simulink library "PhD_Library"  (R2018a)
settings: Solver=VariableStepAuto  StartTime=0.0  StopTime=10.0  RelTol=1e-3
values from neighbouring files (symbols this model uses):
  fn = 60    [Basics_01_Param.m]    (also in FIRs.m = 50; PostSubmission_FreqResp_00_Param.m; XoverRCalc.m)
  Ts_control = 1/20000    (= 5e-05)    [Basics_01_Param.m]    (also in PostSubmission_FreqResp_00_Param.m)
  Ts_PWM = 1/200000    (= 5e-06)    [Basics_01_Param.m]    (also in PostSubmission_FreqResp_00_Param.m)
  Uanp = 1    [Basics_01_Param.m]    (also in PostSubmission_FreqResp_00_Param.m)
undefined symbols (not defined in the file or in its folder): D1, Delta, DiscIntNeverNeededParam, ESS, Iap, PCC, Sn, tctrl, WT
libraries: $bdroot x49, powerlib_meascontrol x39, peTransforms x28, powerlib x18
(part 1 of 3)
settings Model: Creator=daniemot  LastModifiedBy=daniemot

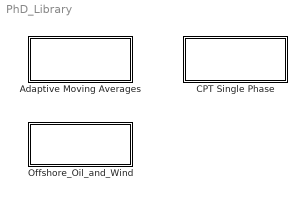
== system PhD_Library ==
  Adaptive Moving Averages : Subsystem
  CPT Single Phase : Subsystem
  Offshore_Oil_and_Wind : Subsystem

== system PhD_Library/Adaptive Moving Averages ==
  AMA with insertion pointer driven buffer : Subsystem  TreatAsAtomicUnit=on  SystemSampleTime=Ts  mask(AMA with insertion pointer driven){NbSize=100, Ts=0.001}
      mask prompts: NbSize "Max number of samples for averaging"; Ts "Sampling time [s]"
      mask help:
      | Adaptive moving average with insertion pointer driven circular buffer
      |
      | Interface
      | Input	x (scalar): signal for averaging
      | 	n (scalar): number of previous samples of the input to be averaged with the current input
      | Output	xavg (scalar): average of the current input and the last n-samples of the input.
      | 	xacc (scalar): internal value sent for accumulation
      | 	xdec (scalar): internal value sent for decumulation
      | Parameters	nmax (scalar): maximum length of the length of the circular buffer
      | 	Ts (scalar): sampling time in [s]
      | Internal circular buffer:
      | 	Insertion pointer: i, always marches forward, x(now) replaces the slot pointed by i
      | 	Retrieval pointer: r, lags i by n samples, zeros the slot once retrieved, allowed to jump backwards, collects all values for decumulation and zeros slots when jumping forward.
      |
      | Prog/rev. semi-history:
      | 	Mota, 2020-11-24: first release
  AMA with lossy buffer : Subsystem  TreatAsAtomicUnit=on  SystemSampleTime=Ts  mask(AMA with a skipping circular buffer.){NbSize=100, Ts=0.001}
      mask prompts: NbSize "Max number of samples for averaging"; Ts "Sampling time [s]"
      mask help:
      | Adaptive moving average built with Matlab's discrete variable time delay
      |
      | Interface
      | Input	x (scalar): signal for averaging
      | 	n (scalar): number of previous samples of the input to be averaged with the current input
      | Output	xavg (scalar): average of the current input and the last n-samples of the input.
      | 	xacc (scalar): internal value sent for accumulation
      | 	xdec (scalar): internal value sent for decumulation
      | Parameters	nmax (scalar): maximum length of the length of the circular buffer
      | 	Ts (scalar): sampling time in [s]
      | Internal circular buffer:
      | 	Matlab's variable discrete time delay
      | 	Skips/double decumulations when n changes
      |
      | Prog/rev. semi-history:
      | 	Mota, 2020-11-24: first release
  AMA with retrieval pointer driven buffer : Subsystem  TreatAsAtomicUnit=on  SystemSampleTime=Ts  mask(AMA with retrieval pointer driven buffer){NbSize=100, Ts=0.001}
      mask prompts: NbSize "Max number of samples for averaging"; Ts "Sampling time [s]"
      mask help:
      | Adaptive moving average with retrieval poitner driven circular buffer
      |
      | Interface
      | Input	x (scalar): signal for averaging
      | 	n (scalar): number of previous samples of the input to be averaged with the current input
      | Output	xavg (scalar): average of the current input and the last n-samples of the input.
      | 	xacc (scalar): internal value sent for accumulation
      | 	xdec (scalar): internal value sent for decumulation
      | Parameters	nmax (scalar): maximum length of the length of the circular buffer
      | 	Ts (scalar): sampling time in [s]
      | Internal circular buffer:
      | 	Retrieval pointer: r, always marches forward, zero the slot after retrieval.
      | 	Insertion pointer: i, marches n slots ahead of r, allowed to jump, sums x(now) to the whichever value present at the insertion slot
      |
      | Prog/rev. semi-history:
      | 	Mota, 2020-11-24: first release
  Subsystem : Subsystem  TreatAsAtomicUnit=on  SystemSampleTime=Ts  mask(HAMA with retrieval pointer driven buffer){NbSize=100, Ts=0.001}
      mask prompts: NbSize "Max number of samples for averaging"; Ts "Sampling time [s]"
      mask help:
      | Hybrid adaptive moving average with three retrieval pointer driven circular buffers.
      |
      | Interface
      | Input	x (scalar): signal for averaging
      | 	n (scalar): number of previous samples of the input to be averaged with the current input
      | Output	xavg (scalar): average of the current input and the last hybrid number of 'n'-samples of the input.
      | 	xavground (scalar): average of the current input and the last round(n)-samples of the input.
      | 	xavgceil (scalar): average of the current input and the last ceil(n)-samples of the input.
      | 	xavgfloor (scalar): average of the current input and the last floor(n)-samples of the input.
      | 	xavgweighed (scalar): average of the current input and the last weighted(n)-samples of the input.
      | Parameters	nmax (scalar): maximum length of the length of the circular buffer
      | 	Ts (scalar): sampling time in [s]
      |
      | Prog/rev. semi-history:
      | 	Mota, 2020-12-08: first release
  WAMA with insertion pointer driven buffer : Subsystem  TreatAsAtomicUnit=on  SystemSampleTime=Ts  mask(WAMA with insertion pointer driven buffer){NbSize=0, Ts=0}
      mask prompts: NbSize "Max number of samples for averaging"; Ts "Sampling time [s]"
      mask help:
      | Adaptive moving average with two insertion pointer driven circular buffers.
      |
      | Interface
      | Input	x (scalar): signal for averaging
      | 	n (scalar): number of previous samples of the input to be averaged with the current input
      | Output	xavg (scalar): weigthed average of the current input and the last 'n'-samples of the input.
      | 	xavgceil (scalar): average of the current input and the last ceil(n)-samples of the input.
      | 	xavgfloor (scalar): average of the current input and the last floor(n)-samples of the input.
      | Parameters	nmax (scalar): maximum length of the length of the circular buffer
      | 	Ts (scalar): sampling time in [s]
      |
      | Prog/rev. semi-history:
      | 	Mota, 2020-11-24: first release
  WAMA with retrieval pointer driven buffers : Subsystem  TreatAsAtomicUnit=on  SystemSampleTime=Ts  mask(WAMA with retrieval pointer driven buffer){NbSize=100, Ts=0.001}
      mask prompts: NbSize "Max number of samples for averaging"; Ts "Sampling time [s]"
      mask help:
      | Adaptive moving average with two retrieval pointer driven circular buffers.
      |
      | Interface
      | Input	x (scalar): signal for averaging
      | 	n (scalar): number of previous samples of the input to be averaged with the current input
      | Output	xavg (scalar): weigthed average of the current input and the last 'n'-samples of the input.
      | 	xavgceil (scalar): average of the current input and the last ceil(n)-samples of the input.
      | 	xavgfloor (scalar): average of the current input and the last floor(n)-samples of the input.
      | Parameters	nmax (scalar): maximum length of the length of the circular buffer
      | 	Ts (scalar): sampling time in [s]
      |
      | Prog/rev. semi-history:
      | 	Mota, 2020-11-24: first release

== system PhD_Library/CPT Single Phase ==
  Single phase CPT Lossy AMA : Subsystem  TreatAsAtomicUnit=on  SystemSampleTime=Ts  mask(Single phase CPT transducer with Skipping AMAs){NbSize=100, Ts=0.001}
      mask prompts: NbSize "Maximum number of samples per period"; Ts "Sampling time [s]"
      mask help:
      | Input	Voltage: v, scalar
      | 	Current: i, scalar
      | 	Frequecy: f, scalar in [Hz]
      | Output	Active power: p
      | 	Active current: ia
      | 	Reactive power: q
      | 	Reactive energy: w
      | 	Reactive current: ir
      | 	Void current: iv
      | 	Integral of the voltage: vint
      | 	Bias of the int. of the volt.: vintbias
      | 	Voltage times current: vi
      | 	Unbiased int. voltage times current: vinthati
      | Parameters	nmax (scalar): maximum length of the length of the circular buffers
      | 	Ts (scalar): sampling time in [s]
      |
      | Prog/rev. semi-history:
      | 	Mota, 2020-11-24: first release
      | 	Mota, 2020-12-08: added voltages and currents to interface
  Single phase CPT Retrieval AMA : Subsystem  TreatAsAtomicUnit=on  SystemSampleTime=Ts  mask(Single Phase CPT Retrieval AMAs){NbSize=100, Ts=0.001}
      mask prompts: NbSize "Maximum number of samples per period"; Ts "Sampling time [s]"
      mask help:
      | Input	Voltage: v, scalar
      | 	Current: i, scalar
      | 	Frequecy: f, scalar in [Hz]
      | Output	Active power: p
      | 	Active current: ia
      | 	Reactive power: q
      | 	Reactive energy: w
      | 	Reactive current: ir
      | 	Void current: iv
      | 	Integral of the voltage: vint
      | 	Bias of the int. of the volt.: vintbias
      | 	Voltage times current: vi
      | 	Unbiased int. voltage times current: vinthati
      | Parameters	nmax (scalar): maximum length of the length of the circular buffers
      | 	Ts (scalar): sampling time in [s]
      |
      | Prog/rev. semi-history:
      | 	Mota, 2020-11-24: first release
      | 	Mota, 2020-12-08: added voltages and currents to interface
  Single phase CPT Retrieval HAMA : Subsystem  TreatAsAtomicUnit=on  SystemSampleTime=Ts  mask{NbSize=100, Ts=0.001}
      mask prompts: NbSize "Maximum number of samples per period"; Ts "Sampling time [s]"
      mask help:
      | Input	Voltage: v, scalar
      | 	Current: i, scalar
      | 	Frequecy: f, scalar in [Hz]
      | Output	Active power: p
      | 	Active current: ia
      | 	Reactive power: q
      | 	Reactive energy: w
      | 	Reactive current: ir
      | 	Void current: iv
      | 	Integral of the voltage: vint
      | 	Bias of the int. of the volt.: vintbias
      | 	Voltage times current: vi
      | 	Unbiased int. voltage times current: vinthati
      | Parameters	nmax (scalar): maximum length of the length of the circular buffers
      | 	Ts (scalar): sampling time in [s]
      |
      | Prog/rev. semi-history:
      | 	Mota, 2020-12-08: first release
  Single phase CPT Retrieval WAMA : Subsystem  TreatAsAtomicUnit=on  SystemSampleTime=Ts  mask(Single phase CPT with Retrieval WAMAs){NbSize=100, Ts=0.001}
      mask prompts: NbSize "Maximum number of samples per period"; Ts "Sampling time [s]"
      mask help:
      | Input	Voltage: v, scalar
      | 	Current: i, scalar
      | 	Frequecy: f, scalar in [Hz]
      | Output	Active power: p
      | 	Active current: ia
      | 	Reactive power: q
      | 	Reactive energy: w
      | 	Reactive current: ir
      | 	Void current: iv
      | 	Integral of the voltage: vint
      | 	Bias of the int. of the volt.: vintbias
      | 	Voltage times current: vi
      | 	Unbiased int. voltage times current: vinthati
      | Parameters	nmax (scalar): maximum length of the length of the circular buffers
      | 	Ts (scalar): sampling time in [s]
      |
      | Prog/rev. semi-history:
      | 	Mota, 2020-11-24: first release
      | 	Mota, 2020-12-08: added voltages and currents to interface

== system PhD_Library/Offshore_Oil_and_Wind ==
  note: WILL MOST LIKELY BE ABANDONED
  Balanced_3_phase_Vsource : Subsystem  mask(Three-phase ideal voltage source){BaseAmp=1, fn=50}
      mask prompts: BaseAmp "Base phase-to-neutral amplitude [V]"; fn "Base frequency [Hz]"
      mask help:
      | Three-phase balanced ideal voltage source with neutral point not connected.
      | The voltage source can be connected in series with others.
      |
      | va [V] = amp_pu*BaseAmp*sin(2*pi*f_pu*fn*time + phase_deg*pi/180)
      | vb [V] = amp_pu*BaseAmp*sin(2*pi*f_pu*fn*time + phase_deg*pi/180 + Ph_b_sign*2*pi/3)
      | vc [V] = amp_pu*BaseAmp*sin(2*pi*f_pu*fn*time + phase_deg*pi/180 + Ph_c_sign*2*pi/3)
      |
      | If Pos1_Neg-1 = 1
      | 	Ph_b_sign = -1
      | 	Ph_c_sign = +1
      |
      | If Pos1_Neg-1 = -1
      | 	Ph_b_sign = +1
      | 	Ph_c_sign = -1
  Digital first order LPF : Subsystem  mask(Digital first order low pass filter){Ts=tctrl, fcutout=fn/2^0.5}
      mask prompts: Ts "Sample times [s]"; fcutout "Cutout frequency [Hz]"
      mask help:
      | Integration with trapezoidal approximation.
      |
      | "Continuous time transfer function":  1/(1 + s T)
      | where T [s] = 1 / (2 * pi * fcutout [Hz]).
      mask Display: fprintf('1/(1 + s T))');
  Idq_Controller : Subsystem  mask(Idq Controller - PI regulator with anti-windup){Ts=Ts_control, fn=fn, Kp=0.4, Ti=0.13, I_ini_d=0.14, I_ini_q=0.07, L=WT.LSC.lf1, PI_max=1.5, PI_min=-1.5, TrafoPhaseComp=0}
      mask prompts: Ts "Sampling time [s]"; fn "Rated frequency: fn [Hz]"; Kp "Proportional gain: Kp [pu]"; Ti "Integral time: Ti [s]"; I_ini_d "Initial value for D integrator [pu]"; I_ini_q "Initial value for Q integrator [pu]"; L "DQ decoupl. inductance: L [pu]"; PI_max "Maximum output [pu]"; PI_min "Minimum output [pu]"; TrafoPhaseComp "Transformer phase compensation [rad]"
      mask help:
      | Idq Controller
      | Discrete PI regulator with forward Euler approximation for the integrator.
      | Transfer function: 	Kp (1 + sTi) / (sTi)
      | The anti-windup freezes the integrator if the unlimited output of the PI goes beyond the limits.
      |
      | Phase compensation for transformer winding: PhaseTrafoComp
  Idq_Decouling_Signs : Subsystem  mask(Idq Controller - PI regulator with anti-windup){Ts=Ts_control, fn=50, Kp=0.4, Ti=0.13, I_ini_d=0.14, I_ini_q=0.07, L=0.3, PI_max=1.5, PI_min=-1.5, TrafoPhaseComp=0}
      mask prompts: Ts "Sampling time [s]"; fn "Rated frequency: fn [Hz]"; Kp "Proportional gain: Kp [pu]"; Ti "Integral time: Ti [s]"; I_ini_d "Initial value for D integrator [pu]"; I_ini_q "Initial value for Q integrator [pu]"; L "DQ decoupl. inductance: L [pu]"; PI_max "Maximum output [pu]"; PI_min "Minimum output [pu]"; TrafoPhaseComp "Transformer phase compensation [rad]"
      mask help:
      | Idq Controller
      | Discrete PI regulator with forward Euler approximation for the integrator.
      | Transfer function: 	Kp (1 + sTi) / (sTi)
      | The anti-windup freezes the integrator if the unlimited output of the PI goes beyond the limits.
      |
      | Phase compensation for transformer winding: PhaseTrafoComp
  LSC_LCL_Trafo : Subsystem  mask(LSC + LCL + Trafo){Sn=WT.Sb, fn=fn, Uhv_ab=WT.ColSys.Ub, Uab=WT.LSC.Ub, lf2=WT.LSC.lf2, rf2=WT.LSC.rf2, Lf1=WT.LSC.Lf1, Rf1=WT.LSC.Rf1, Cf=WT.LSC.Cf, Rc=WT.LSC.Rc}
      mask prompts: Sn "Rated apparent power [VA]"; fn "Rated frequency [Hz]"; Uhv_ab "Trafo HV rated line voltage [V]"; Uab "Trafo LV rated line voltage [V]"; lf2 "Trafo short-circuit inductance, lf2 [pu]"; rf2 "Trafo short-circuit resistance, rf2 [pu]"; Lf1 "Inverter side inductande, Lf1 [H]"; Rf1 "Inverter side parasitic resistance, Rf1 [Ohm]"; Cf "Shunt branch capacitance, Cf [F]"; Rc "Shunt branch damping resistance, Rc [Ohm]"
      mask help:
      | Line side converter + LCL filter + Transformer
      |
      | LSC: switching devices
      | LCL:
      | 	Lf1 + Rf1: inverter side reactor
      | 	Cf + Rc: shunt capacitor and damping resistor
      | 	Lf2 + Rf2: transformer short circuit inductance and resistance
      |
      | Transformer:	Y d1
      | 	HV: Y ungrounded
      | 	LV: delta
      |
      | High resistive grounding on LV side of tranformer (0.001W)
  PI_Kp_Ti_AntiWindup : Subsystem  TreatAsAtomicUnit=on  SystemSampleTime=Ts  mask(PI regulator with anti-windup){Ts=0.001, Kp=10, Ti=1, I_ini=0, PI_max=1, PI_min=-1}
      mask prompts: Ts "Sampling time [s]"; Kp "Proportional gain: Kp [pu]"; Ti "Integral time: Ti [s]"; I_ini "Initial value for the integrator [pu]"; PI_max "Maximum output [pu]"; PI_min "Minimum output [pu]"
      mask help:
      | Discrete PI regulator with forward Euler approximation for the integrator.
      |
      | Transfer function:
      | 	Kp (1 + sTi) / (sTi)
      |
      | The anti-windup freezes the integrator if the unlimited output of the PI goes beyond the limits.
      mask Display: fprintf('Kp(1+1/(sTi))');
  PLL : Subsystem  mask(Matlabs PLL with POS and NEG omega t output){fn=0, Ts=0.00005, Kp_pll=90, Ki_pll=1600, Kd_pll=0, PLL_ini=0}
      mask prompts: fn "Rated frequency [Hz]"; Ts "Sampling time [s]"; Kp_pll "Proportional gain: Kp_pll"; Ki_pll "Integral gain: Ki_pll"; Kd_pll "Derivative gain: Kd_pll"; PLL_ini "PLL initial angle: PLL_ini [degrees]"
  PWM : Subsystem  mask(Scaling of vdq ref and PWM gate generation){fsw=0, Ts=1/200000, Uabp=1000, PWM_Ini_Phase=90}
      mask prompts: fsw "Switching frequency [Hz]"; Ts "Sampling time [s]"; Uabp "Rated peak line voltage [V]"; PWM_Ini_Phase "PWM carrier initial phase [degrees]"
      mask help:
      | Scales vdq_ref by: U_line_peak / Udc
      |
      | Add third harmonic to uabc_ref for overmodulation
  PWM_abc_negwt_acb : Subsystem  mask(Scaling of vdq ref and PWM gate generation){fsw=50, Ts=1/200000, Uabp=1000, PWM_Ini_Phase=90}
      mask prompts: fsw "Switching frequency [Hz]"; Ts "Sampling time [s]"; Uabp "Rated peak line voltage [V]"; PWM_Ini_Phase "PWM carrier initial phase [degrees]"
      mask help:
      | Scales vdq_ref by: U_line_peak / Udc
      |
      | Add third harmonic to uabc_ref for overmodulation
  Scaling_and_PWM : Subsystem  mask(Scaling of vdq ref and PWM gate generation){Ts=Ts_PWM, Uabp=1000, PWM_Ini_Phase=90}
      mask prompts: Ts "Sampling time [s]"; Uabp "Rated peak line voltage [V]"; PWM_Ini_Phase "PWM carrier initial phase [degrees]"
      mask help:
      | Scales vdq_ref by: U_line_peak / Udc
      |
      | Add third harmonic to uabc_ref for overmodulation
  Udc_Controller : Subsystem  mask(Udc Controller - PI regulator with anti-windup){Ts=Ts_control, Kp=WT.LSC.Kp, Ti=WT.LSC.Ti, I_ini=0, PI_max=1.5, PI_min=-1.5}
      mask prompts: Ts "Sampling time [s]"; Kp "Proportional gain: Kp [pu]"; Ti "Integral time: Ti [s]"; I_ini "Initial value for integrator [pu]"; PI_max "Maximum output [pu]"; PI_min "Minimum output [pu]"
      mask help:
      | Udc Controller
      | Discrete PI regulator with forward Euler approximation for the integrator.
      | Transfer function: 	Kp (1 + sTi) / (sTi)
      | The anti-windup freezes the integrator if the unlimited output of the PI goes beyond the limits.
  abc-dq_DDSRF_PLL_Based : Subsystem  mask(abc -> dq based on DDSRF PLL){Ts=Ts_control, fc=fn/2^0.5}
      mask prompts: Ts "Sampling time [s]"; fc "Cutout freq. low pass [Hz]"
      mask help:
      | abc -> dq transducer based on the Decoupled Double Synchronous Reference Frame PLL for Power Converters Control from Rodriguez 2007.
      | The PLL is not implemented, but an output with eq is available for using in a PLL
  abc_dq : Subsystem  mask(abc->dq with Matlab){Ts=0.001, fn=100, fcutoutv=1000, fcutouti=1000, zeta=0.707}
      mask prompts: Ts "Sampling time [s]"; fn "Notch frequency [Hz]"; fcutoutv "Cutout freq. low-pass for vdq meas. [Hz]"; fcutouti "Cutout freq. low-pass for idq meas. [Hz]"; zeta "Zeta for notch filters"
  abc_dq_Rodriguez : Subsystem  mask(abc - dq with double decopupling){Ts=0.00001, fcutout=50/2^0.5}
      mask prompts: Ts "Sampling time [s]"; fcutout "Cutout freq. low pass [Hz]"
      mask help:
      | Double decoupling - Rodriguez
      |
      | The PLL is not implemented, but an output with eq is available for using in a PLL
  abc_dq_with_AMA : Subsystem  mask(abc->dq with Matlab){Ts=0.001, fn=100, fmin=0, fmax=0, fcutoutv=1000, fcutouti=1000}
      mask prompts: Ts "Sampling time [s]"; fn "Rated grid frequency [Hz]"; fmin "Min. acceptable grid freq [Hz]"; fmax "Max. acceptable grid freq [Hz]"; fcutoutv "Cutout freq. low-pass for vdq meas. [Hz]"; fcutouti "Cutout freq. low-pass for idq meas. [Hz]"
  abc_dq_with_PLL : Subsystem  mask(abc->dq with Matlab){Ts=0.001, Kp_pll=90, Ki_pll=1600, Kd_pll=0, PLL_ini=0, fn=50, fcutoutv=1000, fcutouti=1000, zeta=0.7}
      mask prompts: Ts "Sampling time [s]"; Kp_pll "Proportional gain: Kp_pll"; Ki_pll "Integral gain: Ki_pll"; Kd_pll "Derivative gain: Kd_pll"; PLL_ini "PLL initial angle: PLL_ini [degrees]"; fn "Notch frequency [Hz]"; fcutoutv "Cutout freq. low-pass for vdq meas. [Hz]"; fcutouti "Cutout freq. low-pass for idq meas. [Hz]"; zeta "Zeta for all second order filters"
  pqui_Transd_NoZeroSeq : Subsystem  mask(u i p q transducer - No zero sequence){Sn=Sn, Uanp=Uanp, Iap=Iap}
      mask prompts: Sn "Rated three-phase apparent power [VA]"; Uanp "Rated peak phase-to-groud voltage [V]"; Iap "Rated peak line current [A]"
      mask help:
      | Loosely based on Akagi 1984, but with Clarke Transformation for both the current and voltage
      | 	v  = (valpha^2 + vbeta^2)^0.5 / V_phase_peak
      | 	i   = (ialpha^2 + ibeta^2)^0.5 / I_line_peak
      | 	p  = 3/2 * (valpha ialpha +vbeta ibeta) / Sn
      | 	q  = 3/2 * (-valpha ibeta +vbeta ialpha) / Sn
  pqui_Transd_NoZeroSeq_Filter : Subsystem  mask(u i p q transducer - No zero sequence){Ts=0.001, Sn=1000, fn=50, Uanp=1000, Iap=1000, fcutoutvi=1000, fcutoutpq=1000, zeta=0.7}
      mask prompts: Ts "Sampling time [s]"; Sn "Rated three-phase apparent power [VA]"; fn "Rated frequency [Hz]"; Uanp "Rated peak phase-to-groud voltage [V]"; Iap "Rated peak line current [A]"; fcutoutvi "Cutout freq. low-pass for v&i meas. [Hz]"; fcutoutpq "Cutout freq. low-pass for p&q meas. [Hz]"; zeta "Zeta for all second order filters"
      mask help:
      | Loosely based on Akagi 1984, but with Clarke Transformation for both the current and voltage
      | 	v  = (valpha^2 + vbeta^2)^0.5 / V_phase_peak
      | 	i   = (ialpha^2 + ibeta^2)^0.5 / I_line_peak
      | 	p  = 3/2 * (valpha ialpha +vbeta ibeta) / Sn
      | 	q  = 3/2 * (-valpha ibeta +vbeta ialpha) / Sn
      |
      | Second order low-pass filter for all measurements
      |
      | Notch filter at the rated frequency

== system PhD_Library/Adaptive Moving Averages/AMA with insertion pointer driven buffer ==
  In1 : Inport
  In2 : Inport  Port=2
  Constant3 : Constant  Value=NbSize
  MATLAB Function : MATLAB Function  TreatAsAtomicUnit=on
  Out1 : Outport
  Out2 : Outport  Port=2
  Out3 : Outport  Port=3
  wires:
  In2/1 -> MATLAB Function/2(n)  "n"
  MATLAB Function/1(xavg) -> Out1/1  "xavg"
  Constant3/1 -> MATLAB Function/3(Nb)
  MATLAB Function/2(xacc) -> Out2/1  "xacc"
  MATLAB Function/3(xdec) -> Out3/1  "xdec"
  In1/1 -> MATLAB Function/1(x)  "x"

== system PhD_Library/Adaptive Moving Averages/AMA with lossy buffer ==
  x : Inport
  n : Inport  Port=2
  Add1 : Sum
  Add4 : Sum  Inputs=+-
  Constant : Constant
  Delay2 : Delay  DelayLength=1  InitialCondition=0  UseCircularBuffer=on  SampleTime=Ts
  Divide1 : Product  Inputs=*/
  Max : MinMax  Function=max  Inputs=2
  Rounding Function : Rounding  Operator=round
  Variable Integer Delay2 : Delay  DelayLengthSource=Input port  DelayLengthUpperLimit=NbSize  UseCircularBuffer=on  SampleTime=Ts
      settings: InputPortMap=u0,p1
  Zero-Order Hold : ZeroOrderHold  Commented=through  SampleTime=Ts
  Zero-Order Hold1 : ZeroOrderHold  Commented=through  SampleTime=Ts
  xavg : Outport
  xacc : Outport  Port=2
  xdec : Outport  Port=3
  wires:
  n/1 -> Zero-Order Hold1/1  "n"
  x/1 -> Zero-Order Hold/1  "x"
  Divide1/1 -> Add4/1, Variable Integer Delay2/1, xacc/1  "xacc"
  Variable Integer Delay2/1 -> Add4/2, xdec/1  "xdec"
  Constant/1 -> Max/2
  Max/1 -> Variable Integer Delay2/2  "n"
  Add4/1 -> Add1/1  "xavg"
  Add1/1 -> Delay2/1, xavg/1  "xavg"
  Delay2/1 -> Add1/2
  Zero-Order Hold/1 -> Divide1/1
  Zero-Order Hold1/1 -> Rounding Function/1
  Rounding Function/1 -> Divide1/2, Max/1

== system PhD_Library/Adaptive Moving Averages/AMA with retrieval pointer driven buffer ==
  In1 : Inport
  In2 : Inport  Port=2
  Constant3 : Constant  Value=NbSize
  MATLAB Function : MATLAB Function  TreatAsAtomicUnit=on
  Out1 : Outport
  Out2 : Outport  Port=2
  Out3 : Outport  Port=3
  wires:
  MATLAB Function/3(xdec) -> Out3/1  "xdec"
  MATLAB Function/1(xavg) -> Out1/1  "xavg"
  Constant3/1 -> MATLAB Function/3(Nb)
  In1/1 -> MATLAB Function/1(x)  "x"
  In2/1 -> MATLAB Function/2(n)  "n"
  MATLAB Function/2(xacc) -> Out2/1  "xacc"

== system PhD_Library/Adaptive Moving Averages/Subsystem ==
  In1 : Inport
  In2 : Inport  Port=2
  Constant3 : Constant  Value=NbSize
  MATLAB Function : MATLAB Function  TreatAsAtomicUnit=on
  Terminator{,1..3} (4 alike) : Terminator
  Out1 : Outport
  Out3 : Outport  Port=2
  Out4 : Outport  Port=3
  Out2 : Outport  Port=4
  Out5 : Outport  Port=5
  wires:
  MATLAB Function/1(xavg) -> Out1/1  "xavg"
  MATLAB Function/2(xavground) -> Out3/1  "xavground"
  MATLAB Function/3(xavgceil) -> Out4/1  "xavgceil"
  MATLAB Function/4(xavgfloor) -> Out2/1  "xavgfloor"
  MATLAB Function/6(nr) -> Terminator/1  "nr"
  MATLAB Function/7(nf) -> Terminator1/1  "nf"
  MATLAB Function/8(nc) -> Terminator2/1  "nc"
  MATLAB Function/9(changecnt) -> Terminator3/1  "changenc"
  In1/1 -> MATLAB Function/1(x)  "x"
  Constant3/1 -> MATLAB Function/3(Nb)
  In2/1 -> MATLAB Function/2(n)  "n"
  MATLAB Function/5(xavgweigthed) -> Out5/1  "xavgw"

== system PhD_Library/Adaptive Moving Averages/WAMA with insertion pointer driven buffer ==
  In1 : Inport
  In2 : Inport  Port=2
  AMA with insertion pointer driven buffer : $bdroot/Adaptive Moving Averages/AMA with insertion pointer driven buffer  NbSize=NbSize  Ts=Ts
  AMA with insertion pointer driven buffer1 : $bdroot/Adaptive Moving Averages/AMA with insertion pointer driven buffer  NbSize=NbSize  Ts=Ts
  Add : Sum
  Constant : Constant
  Constant1 : Constant
  Floor : Rounding  Operator=ceil
  Floor1 : Rounding
  Max : MinMax  Function=max  Inputs=2
  Product : Product
  Product1 : Product
  Subtract : Sum  Inputs=+-
  Subtract1 : Sum  Inputs=+-+
  Terminator{,1..3} (4 alike) : Terminator
  Out1 : Outport
  Out2 : Outport  Port=2
  Out3 : Outport  Port=3
  wires:
  AMA with insertion pointer driven buffer/1 -> Out2/1, Product/1  "xavgceil"
  AMA with insertion pointer driven buffer/2 -> Terminator/1
  Floor1/1 -> AMA with insertion pointer driven buffer1/2, Subtract1/3, Subtract/2
  Product1/1 -> Add/2
  Subtract/1 -> Product/2
  Product/1 -> Add/1
  Add/1 -> Out1/1  "xavg"
  Subtract1/1 -> Product1/1
  AMA with insertion pointer driven buffer1/2 -> Terminator2/1
  AMA with insertion pointer driven buffer1/3 -> Terminator3/1
  Floor/1 -> AMA with insertion pointer driven buffer/2
  AMA with insertion pointer driven buffer1/1 -> Product1/2, Out3/1  "xavgfloor"
  AMA with insertion pointer driven buffer/3 -> Terminator1/1
  Constant1/1 -> Max/2
  Max/1 -> Floor1/1, Subtract1/2, Subtract/1, Floor/1
  In2/1 -> Max/1  "n"
  Constant/1 -> Subtract1/1
  In1/1 -> AMA with insertion pointer driven buffer1/1, AMA with insertion pointer driven buffer/1  "x"

== system PhD_Library/Adaptive Moving Averages/WAMA with retrieval pointer driven buffers ==
  In1 : Inport
  In2 : Inport  Port=2
  AMA with retrieval pointer driven buffer : $bdroot/Adaptive Moving Averages/AMA with retrieval pointer driven buffer  NbSize=NbSize  Ts=Ts
  AMA with retrieval pointer driven buffer1 : $bdroot/Adaptive Moving Averages/AMA with retrieval pointer driven buffer  NbSize=NbSize  Ts=Ts
  Add : Sum
  Constant : Constant
  Constant1 : Constant
  Floor : Rounding  Operator=ceil
  Floor1 : Rounding
  Max : MinMax  Function=max  Inputs=2
  Product : Product
  Product1 : Product
  Subtract : Sum  Inputs=+-
  Subtract1 : Sum  Inputs=+-+
  Terminator{,1..3} (4 alike) : Terminator
  Out1 : Outport
  Out2 : Outport  Port=2
  Out3 : Outport  Port=3
  wires:
  AMA with retrieval pointer driven buffer/3 -> Terminator1/1
  In1/1 -> AMA with retrieval pointer driven buffer1/1, AMA with retrieval pointer driven buffer/1  "x"
  Floor1/1 -> AMA with retrieval pointer driven buffer1/2, Subtract1/3, Subtract/2
  AMA with retrieval pointer driven buffer/2 -> Terminator/1
  Product1/1 -> Add/2
  Subtract1/1 -> Product1/1
  Add/1 -> Out1/1  "xavg"
  Product/1 -> Add/1
  Subtract/1 -> Product/2
  AMA with retrieval pointer driven buffer/1 -> Out2/1, Product/1  "xavgceil"
  Floor/1 -> AMA with retrieval pointer driven buffer/2
  In2/1 -> Max/1  "n"
  AMA with retrieval pointer driven buffer1/2 -> Terminator2/1
  Constant/1 -> Subtract1/1
  AMA with retrieval pointer driven buffer1/1 -> Product1/2, Out3/1  "xavgfloor"
  AMA with retrieval pointer driven buffer1/3 -> Terminator3/1
  Constant1/1 -> Max/2
  Max/1 -> Floor1/1, Subtract1/2, Subtract/1, Floor/1

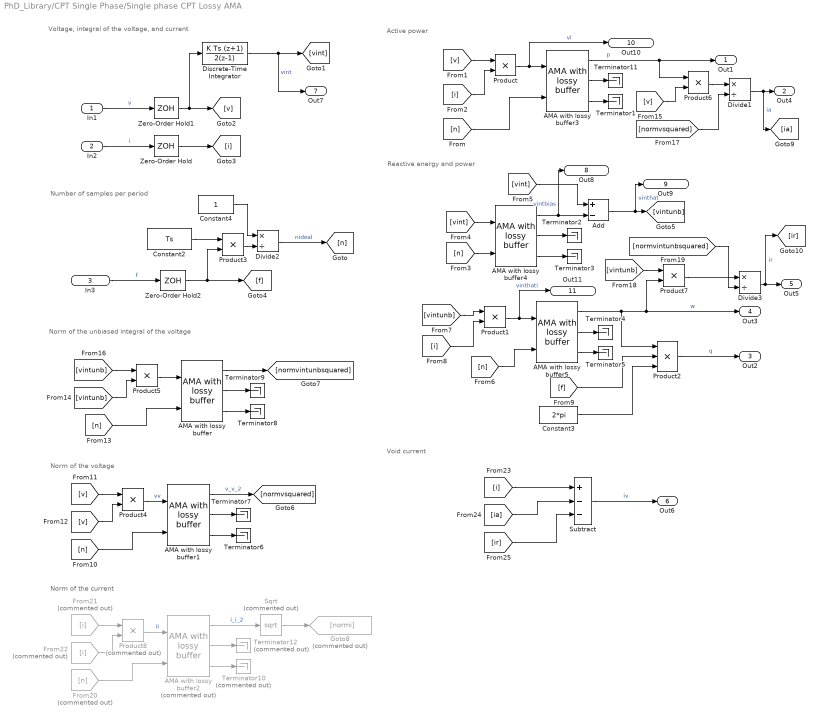
== system PhD_Library/CPT Single Phase/Single phase CPT Lossy AMA ==
  note: Voltage, integral of the voltage, and current
  note: Number of samples per period
  note: Norm of the unbiased integral of the voltage
  note: Norm of the voltage
  note: Active power
  note: Reactive energy and power
  note: Norm of the current
  note: Void current
  In1 : Inport
  In2 : Inport  Port=2
  In3 : Inport  Port=3
  AMA with lossy buffer{,1,3..5} (5 alike) : $bdroot/Adaptive Moving Averages/AMA with lossy buffer  NbSize=NbSize  Ts=Ts
  AMA with lossy buffer2 : $bdroot/Adaptive Moving Averages/AMA with lossy buffer  Commented=on  NbSize=NbSize  Ts=Ts
  Add : Sum  Inputs=+-
  Constant2 : Constant  Value=Ts
  Constant3 : Constant  Value=2*pi
  Constant4 : Constant
  Discrete-Time Integrator : DiscreteIntegrator  IntegratorMethod=Integration: Trapezoidal  SampleTime=Ts  ICPrevOutput=DiscIntNeverNeededParam  ICPrevScaledInput=DiscIntNeverNeededParam
  Divide1 : Product  Inputs=*/
  Divide2 : Product  Inputs=*/
  Divide3 : Product  Inputs=*/
  From20 : From  Commented=on  GotoTag=n
  From21 : From  Commented=on  GotoTag=i
  From22 : From  Commented=on  GotoTag=i
  Goto8 : Goto  Commented=on  GotoTag=normi
  Product{,1,3..7} (7 alike) : Product
  Product2 : Product  Inputs=3
  Product8 : Product  Commented=on
  Sqrt : Sqrt  Commented=on  SaturateOnIntegerOverflow=on
  Subtract : Sum  Inputs=+--
  Terminator{1..9,11} (10 alike) : Terminator
  Terminator10 : Terminator  Commented=on
  Terminator12 : Terminator  Commented=on
  Zero-Order Hold : ZeroOrderHold  SampleTime=Ts
  Zero-Order Hold1 : ZeroOrderHold  SampleTime=Ts
  Zero-Order Hold2 : ZeroOrderHold  SampleTime=Ts
  Out1 : Outport
  Out4 : Outport  Port=2
  Out2 : Outport  Port=3
  Out3 : Outport  Port=4
  Out5 : Outport  Port=5
  Out6 : Outport  Port=6
  Out7 : Outport  Port=7
  Out8 : Outport  Port=8
  Out9 : Outport  Port=9
  Out10 : Outport  Port=10
  Out11 : Outport  Port=11
  wires:
  [n] -> AMA with lossy buffer3/2
  AMA with lossy buffer3/2 -> Terminator11/1
  AMA with lossy buffer3/3 -> Terminator1/1
  Product1/1 -> Out11/1, AMA with lossy buffer5/1  "vinthati"
  AMA with lossy buffer4/1 -> Out8/1, Add/2  "vintbias"
  AMA with lossy buffer4/2 -> Terminator2/1
  [n] -> AMA with lossy buffer4/2
  AMA with lossy buffer5/3 -> Terminator5/1
  AMA with lossy buffer4/3 -> Terminator3/1
  [n] -> AMA with lossy buffer5/2
  AMA with lossy buffer5/1 -> Product7/2, Out3/1, Product2/1  "w"
  [i] -> Product/2
  In1/1 -> Zero-Order Hold1/1  "v"
  In2/1 -> Zero-Order Hold/1  "i"
  [vint] -> Add/1
  Constant4/1 -> Divide2/1
  Divide2/1 -> [n]  "nideal"
  Product3/1 -> Divide2/2
  [v] -> Product/1
  Constant2/1 -> Product3/1
  AMA with lossy buffer5/2 -> Terminator4/1
  [f] -> Product2/2
  Constant3/1 -> Product2/3
  [i] -> Product1/2
  [vint] -> AMA with lossy buffer4/1
  Zero-Order Hold1/1 -> [v], Discrete-Time Integrator/1
  AMA with lossy buffer3/1 -> Product6/1, Out1/1  "p"
  [vintunb] -> Product1/1
  In3/1 -> Zero-Order Hold2/1  "f"
  Product/1 -> Out10/1, AMA with lossy buffer3/1  "vi"
  Zero-Order Hold2/1 -> Product3/2, [f]
  Zero-Order Hold/1 -> [i]
  Product2/1 -> Out2/1  "q"
  Discrete-Time Integrator/1 -> Out7/1, [vint]  "vint"
  Add/1 -> Out9/1, [vintunb]  "vinthat"
  AMA with lossy buffer1/3 -> Terminator6/1
  AMA with lossy buffer1/2 -> Terminator7/1
  AMA with lossy buffer1/1 -> [normvsquared]  "v_v_2"
  [v] -> Product4/1
  [n] -> AMA with lossy buffer1/2
  Product4/1 -> AMA with lossy buffer1/1  "vv"
  [v] -> Product4/2
  [n] -> AMA with lossy buffer/2
  AMA with lossy buffer/2 -> Terminator9/1
  AMA with lossy buffer/1 -> [normvintunbsquared]
  [vintunb] -> Product5/1
  Product5/1 -> AMA with lossy buffer/1
  AMA with lossy buffer/3 -> Terminator8/1
  [vintunb] -> Product5/2
  [v] -> Product6/2
  Product6/1 -> Divide1/1
  [normvsquared] -> Divide1/2
  Divide1/1 -> [ia], Out4/1  "ia"
  [vintunb] -> Product7/1
  Product7/1 -> Divide3/1
  [normvintunbsquared] -> Divide3/2
  Divide3/1 -> [ir], Out5/1  "ir"
  From20/1 -> AMA with lossy buffer2/2
  AMA with lossy buffer2/2 -> Terminator12/1
  AMA with lossy buffer2/1 -> Sqrt/1  "i_i_2"
  From21/1 -> Product8/1
  Product8/1 -> AMA with lossy buffer2/1  "ii"
  AMA with lossy buffer2/3 -> Terminator10/1
  From22/1 -> Product8/2
  Sqrt/1 -> Goto8/1
  [i] -> Subtract/1
  [ia] -> Subtract/2
  [ir] -> Subtract/3
  Subtract/1 -> Out6/1  "iv"

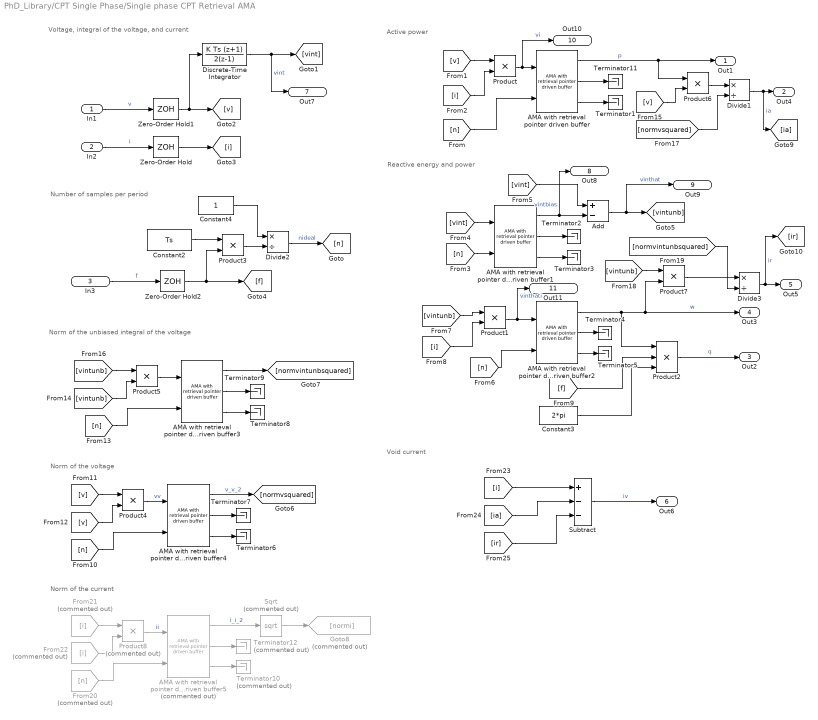
== system PhD_Library/CPT Single Phase/Single phase CPT Retrieval AMA ==
  note: Norm of the voltage
  note: Void current
  note: Active power
  note: Norm of the current
  note: Number of samples per period
  note: Norm of the unbiased integral of the voltage
  note: Reactive energy and power
  note: Voltage, integral of the voltage, and current
  In1 : Inport
  In2 : Inport  Port=2
  In3 : Inport  Port=3
  AMA with retrieval pointer driven buffer{,1..4} (5 alike) : $bdroot/Adaptive Moving Averages/AMA with retrieval pointer driven buffer  NbSize=NbSize  Ts=Ts
  AMA with retrieval pointer driven buffer5 : $bdroot/Adaptive Moving Averages/AMA with retrieval pointer driven buffer  Commented=on  NbSize=NbSize  Ts=Ts
  Add : Sum  Inputs=+-
  Constant2 : Constant  Value=Ts
  Constant3 : Constant  Value=2*pi
  Constant4 : Constant
  Discrete-Time Integrator : DiscreteIntegrator  IntegratorMethod=Integration: Trapezoidal  SampleTime=Ts  ICPrevOutput=DiscIntNeverNeededParam  ICPrevScaledInput=DiscIntNeverNeededParam
  Divide1 : Product  Inputs=*/
  Divide2 : Product  Inputs=*/
  Divide3 : Product  Inputs=*/
  From20 : From  Commented=on  GotoTag=n
  From21 : From  Commented=on  GotoTag=i
  From22 : From  Commented=on  GotoTag=i
  Goto8 : Goto  Commented=on  GotoTag=normi
  Product{,1,3..7} (7 alike) : Product
  Product2 : Product  Inputs=3
  Product8 : Product  Commented=on
  Sqrt : Sqrt  Commented=on  SaturateOnIntegerOverflow=on
  Subtract : Sum  Inputs=+--
  Terminator{1..9,11} (10 alike) : Terminator
  Terminator10 : Terminator  Commented=on
  Terminator12 : Terminator  Commented=on
  Zero-Order Hold : ZeroOrderHold  SampleTime=Ts
  Zero-Order Hold1 : ZeroOrderHold  SampleTime=Ts
  Zero-Order Hold2 : ZeroOrderHold  SampleTime=Ts
  Out1 : Outport
  Out4 : Outport  Port=2
  Out2 : Outport  Port=3
  Out3 : Outport  Port=4
  Out5 : Outport  Port=5
  Out6 : Outport  Port=6
  Out7 : Outport  Port=7
  Out8 : Outport  Port=8
  Out9 : Outport  Port=9
  Out10 : Outport  Port=10
  Out11 : Outport  Port=11
  wires:
  AMA with retrieval pointer driven buffer2/1 -> Product7/2, Out3/1, Product2/1  "w"
  [n] -> AMA with retrieval pointer driven buffer2/2
  [n] -> AMA with retrieval pointer driven buffer1/2
  [i] -> Subtract/1
  AMA with retrieval pointer driven buffer2/3 -> Terminator5/1
  AMA with retrieval pointer driven buffer/2 -> Terminator11/1
  AMA with retrieval pointer driven buffer/1 -> Product6/1, Out1/1  "p"
  Product4/1 -> AMA with retrieval pointer driven buffer4/1  "vv"
  [ia] -> Subtract/2
  [vintunb] -> Product5/1
  Divide3/1 -> [ir], Out5/1  "ir"
  From22/1 -> Product8/2
  Product8/1 -> AMA with retrieval pointer driven buffer5/1  "ii"
  AMA with retrieval pointer driven buffer5/3 -> Terminator10/1
  From21/1 -> Product8/1
  Divide1/1 -> [ia], Out4/1  "ia"
  [normvintunbsquared] -> Divide3/2
  Product7/1 -> Divide3/1
  [n] -> AMA with retrieval pointer driven buffer4/2
  Sqrt/1 -> Goto8/1
  [vintunb] -> Product7/1
  Product1/1 -> Out11/1, AMA with retrieval pointer driven buffer2/1  "vinthati"
  [v] -> Product6/2
  AMA with retrieval pointer driven buffer3/1 -> [normvintunbsquared]
  [normvsquared] -> Divide1/2
  AMA with retrieval pointer driven buffer3/2 -> Terminator9/1
  AMA with retrieval pointer driven buffer2/2 -> Terminator4/1
  AMA with retrieval pointer driven buffer4/1 -> [normvsquared]  "v_v_2"
  [n] -> AMA with retrieval pointer driven buffer3/2
  AMA with retrieval pointer driven buffer4/2 -> Terminator7/1
  Discrete-Time Integrator/1 -> Out7/1, [vint]  "vint"
  Zero-Order Hold/1 -> [i]
  In3/1 -> Zero-Order Hold2/1  "f"
  AMA with retrieval pointer driven buffer/3 -> Terminator1/1
  Zero-Order Hold1/1 -> [v], Discrete-Time Integrator/1
  [vintunb] -> Product1/1
  [i] -> Product1/2
  Constant3/1 -> Product2/3
  [f] -> Product2/2
  [vint] -> Add/1
  [ir] -> Subtract/3
  Constant2/1 -> Product3/1
  Product3/1 -> Divide2/2
  Divide2/1 -> [n]  "nideal"
  [v] -> Product/1
  Zero-Order Hold2/1 -> Product3/2, [f]
  [i] -> Product/2
  In2/1 -> Zero-Order Hold/1  "i"
  In1/1 -> Zero-Order Hold1/1  "v"
  AMA with retrieval pointer driven buffer3/3 -> Terminator8/1
  From20/1 -> AMA with retrieval pointer driven buffer5/2
  Product5/1 -> AMA with retrieval pointer driven buffer3/1
  [n] -> AMA with retrieval pointer driven buffer/2
  [v] -> Product4/1
  [vint] -> AMA with retrieval pointer driven buffer1/1
  AMA with retrieval pointer driven buffer1/2 -> Terminator2/1
  Subtract/1 -> Out6/1  "iv"
  AMA with retrieval pointer driven buffer4/3 -> Terminator6/1
  Product6/1 -> Divide1/1
  AMA with retrieval pointer driven buffer5/1 -> Sqrt/1  "i_i_2"
  Add/1 -> Out9/1, [vintunb]  "vinthat"
  Product/1 -> Out10/1, AMA with retrieval pointer driven buffer/1  "vi"
  AMA with retrieval pointer driven buffer1/3 -> Terminator3/1
  Constant4/1 -> Divide2/1
  [v] -> Product4/2
  [vintunb] -> Product5/2
  Product2/1 -> Out2/1  "q"
  AMA with retrieval pointer driven buffer5/2 -> Terminator12/1
  AMA with retrieval pointer driven buffer1/1 -> Out8/1, Add/2  "vintbias"

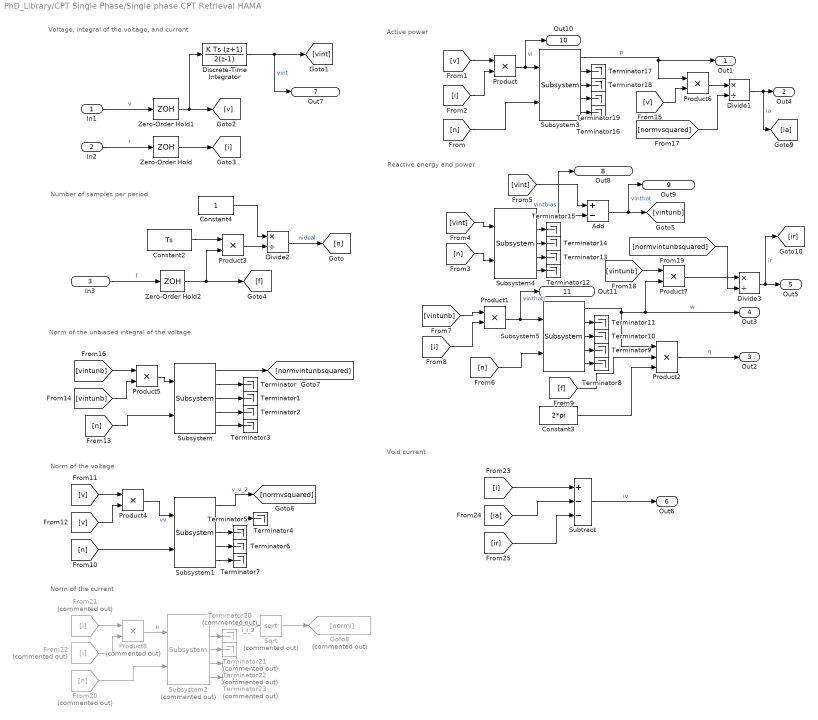
== system PhD_Library/CPT Single Phase/Single phase CPT Retrieval HAMA ==
  note: Void current
  note: Number of samples per period
  note: Norm of the voltage
  note: Voltage, integral of the voltage, and current
  note: Reactive energy and power
  note: Active power
  note: Norm of the current
  note: Norm of the unbiased integral of the voltage
  In1 : Inport
  In2 : Inport  Port=2
  In3 : Inport  Port=3
  Add : Sum  Inputs=+-
  Constant2 : Constant  Value=Ts
  Constant3 : Constant  Value=2*pi
  Constant4 : Constant
  Discrete-Time Integrator : DiscreteIntegrator  IntegratorMethod=Integration: Trapezoidal  SampleTime=Ts  ICPrevOutput=DiscIntNeverNeededParam  ICPrevScaledInput=DiscIntNeverNeededParam
  Divide1 : Product  Inputs=*/
  Divide2 : Product  Inputs=*/
  Divide3 : Product  Inputs=*/
  From20 : From  Commented=on  GotoTag=n
  From21 : From  Commented=on  GotoTag=i
  From22 : From  Commented=on  GotoTag=i
  Goto8 : Goto  Commented=on  GotoTag=normi
  Product{,1,3..7} (7 alike) : Product
  Product2 : Product  Inputs=3
  Product8 : Product  Commented=on
  Sqrt : Sqrt  Commented=on  SaturateOnIntegerOverflow=on
  Subsystem{,1,3..5} (5 alike) : $bdroot/Adaptive Moving Averages/Subsystem  NbSize=NbSize  Ts=Ts
  Subsystem2 : $bdroot/Adaptive Moving Averages/Subsystem  Commented=on  NbSize=NbSize  Ts=Ts
  Subtract : Sum  Inputs=+--
  Terminator{,1..19} (20 alike) : Terminator
  Terminator{20..23} (4 alike) : Terminator  Commented=on
  Zero-Order Hold : ZeroOrderHold  SampleTime=Ts
  Zero-Order Hold1 : ZeroOrderHold  SampleTime=Ts
  Zero-Order Hold2 : ZeroOrderHold  SampleTime=Ts
  Out1 : Outport
  Out4 : Outport  Port=2
  Out2 : Outport  Port=3
  Out3 : Outport  Port=4
  Out5 : Outport  Port=5
  Out6 : Outport  Port=6
  Out7 : Outport  Port=7
  Out8 : Outport  Port=8
  Out9 : Outport  Port=9
  Out10 : Outport  Port=10
  Out11 : Outport  Port=11
  wires:
  Product6/1 -> Divide1/1
  [i] -> Product/2
  Product3/1 -> Divide2/2
  Product7/1 -> Divide3/1
  [ia] -> Subtract/2
  [f] -> Product2/2
  Divide3/1 -> [ir], Out5/1  "ir"
  Subsystem2/1 -> Sqrt/1  "i_i_2"
  Product8/1 -> Subsystem2/1  "ii"
  [v] -> Product4/1
  Subtract/1 -> Out6/1  "iv"
  In2/1 -> Zero-Order Hold/1  "i"
  In1/1 -> Zero-Order Hold1/1  "v"
  [v] -> Product/1
  [v] -> Product4/2
  [n] -> Subsystem/2
  [vint] -> Add/1
  Add/1 -> Out9/1, [vintunb]  "vinthat"
  From21/1 -> Product8/1
  Subsystem4/1 -> Out8/1, Add/2  "vintbias"
  Zero-Order Hold2/1 -> Product3/2, [f]
  [ir] -> Subtract/3
  Divide2/1 -> [n]  "nideal"
  Product1/1 -> Subsystem5/1, Out11/1  "vinthati"
  Zero-Order Hold/1 -> [i]
  Divide1/1 -> [ia], Out4/1  "ia"
  [vintunb] -> Product7/1
  Product2/1 -> Out2/1  "q"
  Constant3/1 -> Product2/3
  From22/1 -> Product8/2
  [vintunb] -> Product5/1
  [normvintunbsquared] -> Divide3/2
  Discrete-Time Integrator/1 -> Out7/1, [vint]  "vint"
  [vintunb] -> Product5/2
  [i] -> Subtract/1
  Product5/1 -> Subsystem/1
  [vintunb] -> Product1/1
  Subsystem1/1 -> [normvsquared]  "v_v_2"
  Product/1 -> Subsystem3/1, Out10/1  "vi"
  [v] -> Product6/2
  Constant2/1 -> Product3/1
  [i] -> Product1/2
  Product4/1 -> Subsystem1/1  "vv"
  [n] -> Subsystem1/2
  Subsystem5/1 -> Product2/1, Product7/2, Out3/1  "w"
  [normvsquared] -> Divide1/2
  Zero-Order Hold1/1 -> [v], Discrete-Time Integrator/1
  In3/1 -> Zero-Order Hold2/1  "f"
  Constant4/1 -> Divide2/1
  Subsystem/1 -> [normvintunbsquared]
  Sqrt/1 -> Goto8/1
  Subsystem3/1 -> Product6/1, Out1/1  "p"
  From20/1 -> Subsystem2/2
  [n] -> Subsystem3/2
  [vint] -> Subsystem4/1
  [n] -> Subsystem4/2
  [n] -> Subsystem5/2
  Subsystem/2 -> Terminator/1
  Subsystem/3 -> Terminator1/1
  Subsystem/4 -> Terminator2/1
  Subsystem/5 -> Terminator3/1
  Subsystem1/2 -> Terminator4/1
  Subsystem1/3 -> Terminator5/1
  Subsystem1/4 -> Terminator6/1
  Subsystem1/5 -> Terminator7/1
  Subsystem5/5 -> Terminator8/1
  Subsystem5/4 -> Terminator9/1
  Subsystem5/3 -> Terminator10/1
  Subsystem5/2 -> Terminator11/1
  Subsystem4/5 -> Terminator12/1
  Subsystem4/4 -> Terminator13/1
  Subsystem4/3 -> Terminator14/1
  Subsystem4/2 -> Terminator15/1
  Subsystem3/5 -> Terminator16/1
  Subsystem3/2 -> Terminator17/1
  Subsystem3/3 -> Terminator18/1
  Subsystem3/4 -> Terminator19/1
  Subsystem2/2 -> Terminator20/1
  Subsystem2/3 -> Terminator21/1
  Subsystem2/4 -> Terminator22/1
  Subsystem2/5 -> Terminator23/1

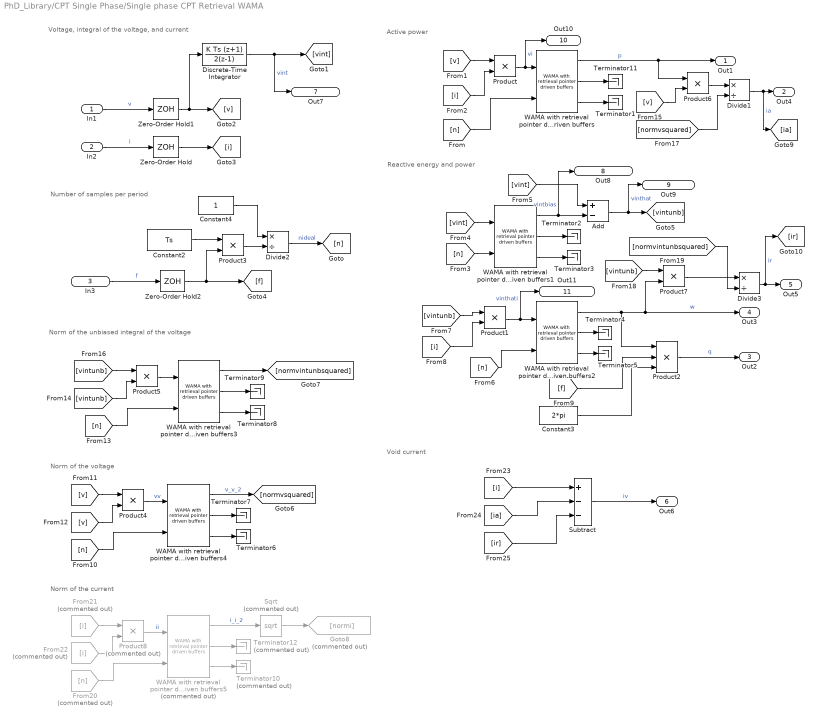
== system PhD_Library/CPT Single Phase/Single phase CPT Retrieval WAMA ==
  note: Voltage, integral of the voltage, and current
  note: Number of samples per period
  note: Reactive energy and power
  note: Active power
  note: Norm of the voltage
  note: Norm of the unbiased integral of the voltage
  note: Norm of the current
  note: Void current
  In1 : Inport
  In2 : Inport  Port=2
  In3 : Inport  Port=3
  Add : Sum  Inputs=+-
  Constant2 : Constant  Value=Ts
  Constant3 : Constant  Value=2*pi
  Constant4 : Constant
  Discrete-Time Integrator : DiscreteIntegrator  IntegratorMethod=Integration: Trapezoidal  SampleTime=Ts  ICPrevOutput=DiscIntNeverNeededParam  ICPrevScaledInput=DiscIntNeverNeededParam
  Divide1 : Product  Inputs=*/
  Divide2 : Product  Inputs=*/
  Divide3 : Product  Inputs=*/
  From20 : From  Commented=on  GotoTag=n
  From21 : From  Commented=on  GotoTag=i
  From22 : From  Commented=on  GotoTag=i
  Goto8 : Goto  Commented=on  GotoTag=normi
  Product{,1,3..7} (7 alike) : Product
  Product2 : Product  Inputs=3
  Product8 : Product  Commented=on
  Sqrt : Sqrt  Commented=on  SaturateOnIntegerOverflow=on
  Subtract : Sum  Inputs=+--
  Terminator{1..9,11} (10 alike) : Terminator
  Terminator10 : Terminator  Commented=on
  Terminator12 : Terminator  Commented=on
  WAMA with retrieval pointer driven buffers{,1..4} (5 alike) : $bdroot/Adaptive Moving Averages/WAMA with retrieval pointer driven buffers  NbSize=NbSize  Ts=Ts
  WAMA with retrieval pointer driven buffers5 : $bdroot/Adaptive Moving Averages/WAMA with retrieval pointer driven buffers  Commented=on  NbSize=NbSize  Ts=Ts
  Zero-Order Hold : ZeroOrderHold  SampleTime=Ts
  Zero-Order Hold1 : ZeroOrderHold  SampleTime=Ts
  Zero-Order Hold2 : ZeroOrderHold  SampleTime=Ts
  Out1 : Outport
  Out4 : Outport  Port=2
  Out2 : Outport  Port=3
  Out3 : Outport  Port=4
  Out5 : Outport  Port=5
  Out6 : Outport  Port=6
  Out7 : Outport  Port=7
  Out8 : Outport  Port=8
  Out9 : Outport  Port=9
  Out10 : Outport  Port=10
  Out11 : Outport  Port=11
  wires:
  Discrete-Time Integrator/1 -> Out7/1, [vint]  "vint"
  In3/1 -> Zero-Order Hold2/1  "f"
  Zero-Order Hold1/1 -> [v], Discrete-Time Integrator/1
  [i] -> Subtract/1
  WAMA with retrieval pointer driven buffers3/1 -> [normvintunbsquared]
  Product5/1 -> WAMA with retrieval pointer driven buffers3/1
  WAMA with retrieval pointer driven buffers3/2 -> Terminator9/1
  WAMA with retrieval pointer driven buffers3/3 -> Terminator8/1
  Product4/1 -> WAMA with retrieval pointer driven buffers4/1  "vv"
  WAMA with retrieval pointer driven buffers4/3 -> Terminator6/1
  WAMA with retrieval pointer driven buffers4/2 -> Terminator7/1
  WAMA with retrieval pointer driven buffers4/1 -> [normvsquared]  "v_v_2"
  [n] -> WAMA with retrieval pointer driven buffers4/2
  [vint] -> WAMA with retrieval pointer driven buffers1/1
  WAMA with retrieval pointer driven buffers5/3 -> Terminator10/1
  WAMA with retrieval pointer driven buffers1/2 -> Terminator2/1
  WAMA with retrieval pointer driven buffers/2 -> Terminator11/1
  WAMA with retrieval pointer driven buffers/3 -> Terminator1/1
  WAMA with retrieval pointer driven buffers2/2 -> Terminator4/1
  Product1/1 -> Out11/1, WAMA with retrieval pointer driven buffers2/1  "vinthati"
  [v] -> Product6/2
  WAMA with retrieval pointer driven buffers2/1 -> Product7/2, Out3/1, Product2/1  "w"
  Product/1 -> Out10/1, WAMA with retrieval pointer driven buffers/1  "vi"
  [vintunb] -> Product7/1
  [normvsquared] -> Divide1/2
  [normvintunbsquared] -> Divide3/2
  Divide1/1 -> [ia], Out4/1  "ia"
  Zero-Order Hold/1 -> [i]
  [vint] -> Add/1
  Constant3/1 -> Product2/3
  [i] -> Product1/2
  [vintunb] -> Product1/1
  Constant2/1 -> Product3/1
  [vintunb] -> Product5/1
  [ir] -> Subtract/3
  From22/1 -> Product8/2
  [n] -> WAMA with retrieval pointer driven buffers2/2
  WAMA with retrieval pointer driven buffers5/2 -> Terminator12/1
  Zero-Order Hold2/1 -> Product3/2, [f]
  Product7/1 -> Divide3/1
  WAMA with retrieval pointer driven buffers1/3 -> Terminator3/1
  Sqrt/1 -> Goto8/1
  Divide2/1 -> [n]  "nideal"
  WAMA with retrieval pointer driven buffers5/1 -> Sqrt/1  "i_i_2"
  Constant4/1 -> Divide2/1
  Product2/1 -> Out2/1  "q"
  [n] -> WAMA with retrieval pointer driven buffers3/2
  Product3/1 -> Divide2/2
  [n] -> WAMA with retrieval pointer driven buffers/2
  From20/1 -> WAMA with retrieval pointer driven buffers5/2
  [vintunb] -> Product5/2
  [v] -> Product4/2
  Product8/1 -> WAMA with retrieval pointer driven buffers5/1  "ii"
  Product6/1 -> Divide1/1
  WAMA with retrieval pointer driven buffers1/1 -> Out8/1, Add/2  "vintbias"
  Add/1 -> Out9/1, [vintunb]  "vinthat"
  [f] -> Product2/2
  In1/1 -> Zero-Order Hold1/1  "v"
  From21/1 -> Product8/1
  WAMA with retrieval pointer driven buffers/1 -> Product6/1, Out1/1  "p"
  Subtract/1 -> Out6/1  "iv"
  [i] -> Product/2
  In2/1 -> Zero-Order Hold/1  "i"
  [n] -> WAMA with retrieval pointer driven buffers1/2
  Divide3/1 -> [ir], Out5/1  "ir"
  [v] -> Product4/1
  WAMA with retrieval pointer driven buffers2/3 -> Terminator5/1
  [v] -> Product/1
  [ia] -> Subtract/2

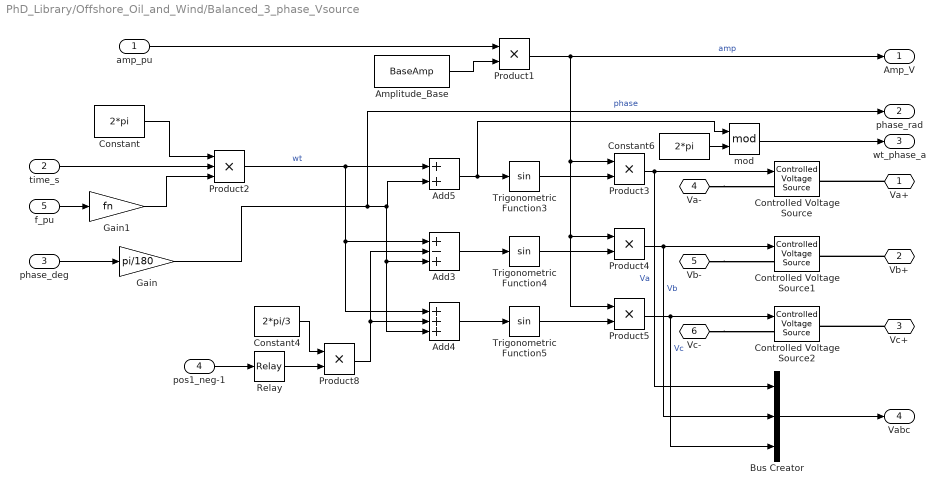
== system PhD_Library/Offshore_Oil_and_Wind/Balanced_3_phase_Vsource ==
  amp_pu : Inport
  time_s : Inport  Port=2
  phase_deg : Inport  Port=3
  pos1_neg-1 : Inport  Port=4
  f_pu : Inport  Port=5
  Add3 : Sum  Inputs=+-+
  Add4 : Sum  Inputs=+++
  Add5 : Sum
  Amplitude_Base : Constant  Value=BaseAmp
  Bus Creator : BusCreator  Inputs=3
  Constant : Constant  Value=2*pi
  Constant4 : Constant  Value=2*pi/3
  Constant6 : Constant  Value=2*pi
  Controlled Voltage Source : powerlib/Electrical Sources/Controlled Voltage Source  Initialize=off  Source_Type=AC  Amplitude=ESS.LSC.Ub*(2/3)^0.5  Phase=0  Frequency=PCC.fn  Measurements=None
  Controlled Voltage Source1 : powerlib/Electrical Sources/Controlled Voltage Source  Initialize=off  Source_Type=AC  Amplitude=ESS.LSC.Ub*(2/3)^0.5  Phase=-120  Frequency=PCC.fn  Measurements=None
  Controlled Voltage Source2 : powerlib/Electrical Sources/Controlled Voltage Source  Initialize=off  Source_Type=AC  Amplitude=ESS.LSC.Ub*(2/3)^0.5  Phase=120  Frequency=PCC.fn  Measurements=None
  Gain : Gain  Gain=pi/180
  Gain1 : Gain  Gain=fn
  Product{1,3..5,8} (5 alike) : Product
  Product2 : Product  Inputs=3
  Relay : Relay  OnSwitchValue=0  OffSwitchValue=-0.1  OffOutputValue=-1
  Trigonometric Function3 : Trigonometry
  Trigonometric Function4 : Trigonometry
  Trigonometric Function5 : Trigonometry
  mod : Math  Operator=mod  SaturateOnIntegerOverflow=on
  Va+ : PMIOPort  Side=Right
  Vb+ : PMIOPort  Port=2  Side=Right
  Vc+ : PMIOPort  Port=3  Side=Right
  Va- : PMIOPort  Port=4  Side=Right
  Vb- : PMIOPort  Port=5  Side=Right
  Vc- : PMIOPort  Port=6  Side=Right
  Amp_V : Outport
  phase_rad : Outport  Port=2
  wt_phase_a : Outport  Port=3
  Vabc : Outport  Port=4
  wires:
  Add4/1 -> Trigonometric Function5/1
  Gain/1 -> phase_rad/1, Add4/3, Add3/3, Add5/2  "phase"
  Add3/1 -> Trigonometric Function4/1
  pos1_neg-1/1 -> Relay/1
  Product3/1 -> Bus Creator/1, Controlled Voltage Source/1  "Va"
  amp_pu/1 -> Product1/1
  Product8/1 -> Add3/2, Add4/2
  Product5/1 -> Bus Creator/3, Controlled Voltage Source2/1  "Vc"
  Product4/1 -> Bus Creator/2, Controlled Voltage Source1/1  "Vb"
  Amplitude_Base/1 -> Product1/2
  Constant4/1 -> Product8/1
  Product1/1 -> Product5/1, Product4/1, Product3/1, Amp_V/1  "amp"
  Relay/1 -> Product8/2
  Trigonometric Function3/1 -> Product3/2
  Product2/1 -> Add5/1, Add4/1, Add3/1  "wt"
  Trigonometric Function5/1 -> Product5/2
  Add5/1 -> mod/1, Trigonometric Function3/1
  Trigonometric Function4/1 -> Product4/2
  phase_deg/1 -> Gain/1
  time_s/1 -> Product2/2
  Constant/1 -> Product2/1
  f_pu/1 -> Gain1/1
  Gain1/1 -> Product2/3
  Bus Creator/1 -> Vabc/1
  Constant6/1 -> mod/2
  mod/1 -> wt_phase_a/1
  connections:
  Vb+/RConn1 -- Controlled Voltage Source1/RConn1
  Vc+/RConn1 -- Controlled Voltage Source2/RConn1
  Va+/RConn1 -- Controlled Voltage Source/RConn1
  Va-/RConn1 -- Controlled Voltage Source/LConn1
  Vb-/RConn1 -- Controlled Voltage Source1/LConn1
  Vc-/RConn1 -- Controlled Voltage Source2/LConn1

== system PhD_Library/Offshore_Oil_and_Wind/Digital first order LPF ==
  in : Inport
  Add7 : Sum  Inputs=+-
  Discrete-Time Integrator : DiscreteIntegrator  IntegratorMethod=Integration: Trapezoidal  SampleTime=Ts  ICPrevOutput=DiscIntNeverNeededParam  ICPrevScaledInput=DiscIntNeverNeededParam
  Gain6 : Gain  Gain=2*pi*fcutout
  Rate Transition3 : RateTransition  OutPortSampleTime=Ts
  out : Outport
  wires:
  Add7/1 -> Gain6/1
  Discrete-Time Integrator/1 -> out/1, Add7/2
  in/1 -> Rate Transition3/1
  Gain6/1 -> Discrete-Time Integrator/1
  Rate Transition3/1 -> Add7/1
